simulink model "gm_soc_dvbs2_fpga"  (R2025b)
settings: Solver=VariableStepAuto  StartTime=0.0  StopTime=10.0  RelTol=1e-3
InitFcn:
  | soc_dvbs2_init;
undefined symbols (not defined in the file or in its folder): Add, coefficientsLog, coefficientsSqrt1, coefficientsSqrt2, dataBits, Deinterleaver, designMultirateFIR, noisePow, Shift, Short, soc_dvbs2_designFIRFilter, soc_dvbs2_txPacketBits, syncWord, txDataOut, txFiltCoeff, XData
libraries: simulink x304, hdlsllib x265, dspsigops x15, dsphdlfiltering2 x8, hdlmdlgenlib x6, dsphdlsigops2 x5, commseqgen3 x5, dsphdlmathfun2 x3, hwlogicconnlib x2, whdledac x2, commhdlcrc x2, whdlutilities x1
(part 32 of 36)

== system gm_soc_dvbs2_fpga/DVBS2/DVBS2 TxRx/DVB-S2 HDL Receiver/Synchronizer and PL Header Decoder/PL Header Recovery/PL Header Decoder/ML Decoder/Get Min Index/For Each Subsystem_instance29 ==
  note: For Each
  valueIn : Inport  OutDataTypeStr=fixdt(1, 25, 15)  PortDimensions=[2]  SampleTime=2.5e-07
  idxIn : Inport  Port=2  OutDataTypeStr=fixdt(0, 6, 0)  PortDimensions=[2]  SampleTime=2.5e-07
  Delay{1..9} (9 alike) : Delay  DelayLength=double(1)  InitialCondition=0  SampleTime=2.5e-07
  Relational Operator : RelationalOperator  Operator=<  OutDataTypeStr=boolean  SampleTime=2.5e-07  InputSameDT=off
  Switch : Switch  Criteria=u2 ~= 0  Threshold="fi(0,0,1,0,\"hex\",\"0\")"  OutDataTypeStr=fixdt(1, 25, 15)  SampleTime=2.5e-07  SaturateOnIntegerOverflow=off  InputSameDT=off
  Switch1 : Switch  Criteria=u2 ~= 0  Threshold="fi(0,0,1,0,\"hex\",\"0\")"  OutDataTypeStr=fixdt(0, 6, 0)  SampleTime=2.5e-07  SaturateOnIntegerOverflow=off  InputSameDT=off
  t : Demux  Outputs=2
  t1 : Demux  Outputs=2
  ValueOut : Outport  SampleTime=2.5e-07
  idxOut : Outport  Port=2  SampleTime=2.5e-07
  wires:
  Delay8/1 -> ValueOut/1
  valueIn/1 -> Delay3/1
  idxIn/1 -> Delay1/1
  t/1 -> Delay6/1
  Switch1/1 -> Delay9/1
  t1/1 -> Relational Operator/1, Delay4/1
  Delay1/1 -> t/1
  Delay3/1 -> t1/1
  t/2 -> Delay7/1
  Delay4/1 -> Switch/1
  t1/2 -> Relational Operator/2, Delay5/1
  Relational Operator/1 -> Delay2/1
  Delay5/1 -> Switch/3
  Delay6/1 -> Switch1/1
  Delay7/1 -> Switch1/3
  Delay2/1 -> Switch/2, Switch1/2
  Switch/1 -> Delay8/1
  Delay9/1 -> idxOut/1

== system gm_soc_dvbs2_fpga/DVBS2/DVBS2 TxRx/DVB-S2 HDL Receiver/Synchronizer and PL Header Decoder/PL Header Recovery/PL Header Decoder/ML Decoder/Get Min Index/For Each Subsystem_instance3 ==
  note: For Each
  valueIn : Inport  OutDataTypeStr=fixdt(1, 25, 15)  PortDimensions=[2]  SampleTime=2.5e-07
  idxIn : Inport  Port=2  OutDataTypeStr=fixdt(0, 6, 0)  PortDimensions=[2]  SampleTime=2.5e-07
  Delay{1..9} (9 alike) : Delay  DelayLength=double(1)  InitialCondition=0  SampleTime=2.5e-07
  Relational Operator : RelationalOperator  Operator=<  OutDataTypeStr=boolean  SampleTime=2.5e-07  InputSameDT=off
  Switch : Switch  Criteria=u2 ~= 0  Threshold="fi(0,0,1,0,\"hex\",\"0\")"  OutDataTypeStr=fixdt(1, 25, 15)  SampleTime=2.5e-07  SaturateOnIntegerOverflow=off  InputSameDT=off
  Switch1 : Switch  Criteria=u2 ~= 0  Threshold="fi(0,0,1,0,\"hex\",\"0\")"  OutDataTypeStr=fixdt(0, 6, 0)  SampleTime=2.5e-07  SaturateOnIntegerOverflow=off  InputSameDT=off
  t : Demux  Outputs=2
  t1 : Demux  Outputs=2
  ValueOut : Outport  SampleTime=2.5e-07
  idxOut : Outport  Port=2  SampleTime=2.5e-07
  wires:
  Delay8/1 -> ValueOut/1
  valueIn/1 -> Delay3/1
  idxIn/1 -> Delay1/1
  t/1 -> Delay6/1
  Switch1/1 -> Delay9/1
  t1/1 -> Delay4/1, Relational Operator/1
  Delay1/1 -> t/1
  Delay3/1 -> t1/1
  t/2 -> Delay7/1
  t1/2 -> Relational Operator/2, Delay5/1
  Relational Operator/1 -> Delay2/1
  Delay5/1 -> Switch/3
  Delay6/1 -> Switch1/1
  Delay7/1 -> Switch1/3
  Delay2/1 -> Switch/2, Switch1/2
  Delay4/1 -> Switch/1
  Switch/1 -> Delay8/1
  Delay9/1 -> idxOut/1

== system gm_soc_dvbs2_fpga/DVBS2/DVBS2 TxRx/DVB-S2 HDL Receiver/Synchronizer and PL Header Decoder/PL Header Recovery/PL Header Decoder/ML Decoder/Get Min Index/For Each Subsystem_instance30 ==
  note: For Each
  valueIn : Inport  OutDataTypeStr=fixdt(1, 25, 15)  PortDimensions=[2]  SampleTime=2.5e-07
  idxIn : Inport  Port=2  OutDataTypeStr=fixdt(0, 6, 0)  PortDimensions=[2]  SampleTime=2.5e-07
  Delay{1..9} (9 alike) : Delay  DelayLength=double(1)  InitialCondition=0  SampleTime=2.5e-07
  Relational Operator : RelationalOperator  Operator=<  OutDataTypeStr=boolean  SampleTime=2.5e-07  InputSameDT=off
  Switch : Switch  Criteria=u2 ~= 0  Threshold="fi(0,0,1,0,\"hex\",\"0\")"  OutDataTypeStr=fixdt(1, 25, 15)  SampleTime=2.5e-07  SaturateOnIntegerOverflow=off  InputSameDT=off
  Switch1 : Switch  Criteria=u2 ~= 0  Threshold="fi(0,0,1,0,\"hex\",\"0\")"  OutDataTypeStr=fixdt(0, 6, 0)  SampleTime=2.5e-07  SaturateOnIntegerOverflow=off  InputSameDT=off
  t : Demux  Outputs=2
  t1 : Demux  Outputs=2
  ValueOut : Outport  SampleTime=2.5e-07
  idxOut : Outport  Port=2  SampleTime=2.5e-07
  wires:
  valueIn/1 -> Delay3/1
  idxIn/1 -> Delay1/1
  Delay9/1 -> idxOut/1
  Delay1/1 -> t/1
  Delay3/1 -> t1/1
  t/1 -> Delay6/1
  t1/1 -> Relational Operator/1, Delay4/1
  t/2 -> Delay7/1
  t1/2 -> Relational Operator/2, Delay5/1
  Relational Operator/1 -> Delay2/1
  Delay5/1 -> Switch/3
  Delay6/1 -> Switch1/1
  Switch1/1 -> Delay9/1
  Delay7/1 -> Switch1/3
  Delay2/1 -> Switch1/2, Switch/2
  Delay4/1 -> Switch/1
  Delay8/1 -> ValueOut/1
  Switch/1 -> Delay8/1

== system gm_soc_dvbs2_fpga/DVBS2/DVBS2 TxRx/DVB-S2 HDL Receiver/Synchronizer and PL Header Decoder/PL Header Recovery/PL Header Decoder/ML Decoder/Get Min Index/For Each Subsystem_instance31 ==
  note: For Each
  valueIn : Inport  OutDataTypeStr=fixdt(1, 25, 15)  PortDimensions=[2]  SampleTime=2.5e-07
  idxIn : Inport  Port=2  OutDataTypeStr=fixdt(0, 6, 0)  PortDimensions=[2]  SampleTime=2.5e-07
  Delay{1..9} (9 alike) : Delay  DelayLength=double(1)  InitialCondition=0  SampleTime=2.5e-07
  Relational Operator : RelationalOperator  Operator=<  OutDataTypeStr=boolean  SampleTime=2.5e-07  InputSameDT=off
  Switch : Switch  Criteria=u2 ~= 0  Threshold="fi(0,0,1,0,\"hex\",\"0\")"  OutDataTypeStr=fixdt(1, 25, 15)  SampleTime=2.5e-07  SaturateOnIntegerOverflow=off  InputSameDT=off
  Switch1 : Switch  Criteria=u2 ~= 0  Threshold="fi(0,0,1,0,\"hex\",\"0\")"  OutDataTypeStr=fixdt(0, 6, 0)  SampleTime=2.5e-07  SaturateOnIntegerOverflow=off  InputSameDT=off
  t : Demux  Outputs=2
  t1 : Demux  Outputs=2
  ValueOut : Outport  SampleTime=2.5e-07
  idxOut : Outport  Port=2  SampleTime=2.5e-07
  wires:
  Delay8/1 -> ValueOut/1
  valueIn/1 -> Delay3/1
  Delay1/1 -> t/1
  Switch1/1 -> Delay9/1
  t1/1 -> Relational Operator/1, Delay4/1
  Delay3/1 -> t1/1
  idxIn/1 -> Delay1/1
  Relational Operator/1 -> Delay2/1
  t1/2 -> Delay5/1, Relational Operator/2
  Delay4/1 -> Switch/1
  t/1 -> Delay6/1
  t/2 -> Delay7/1
  Delay5/1 -> Switch/3
  Delay2/1 -> Switch/2, Switch1/2
  Delay6/1 -> Switch1/1
  Delay7/1 -> Switch1/3
  Switch/1 -> Delay8/1
  Delay9/1 -> idxOut/1

== system gm_soc_dvbs2_fpga/DVBS2/DVBS2 TxRx/DVB-S2 HDL Receiver/Synchronizer and PL Header Decoder/PL Header Recovery/PL Header Decoder/ML Decoder/Get Min Index/For Each Subsystem_instance32 ==
  note: For Each
  valueIn : Inport  OutDataTypeStr=fixdt(1, 25, 15)  PortDimensions=[2]  SampleTime=2.5e-07
  idxIn : Inport  Port=2  OutDataTypeStr=fixdt(0, 6, 0)  PortDimensions=[2]  SampleTime=2.5e-07
  Delay{1..9} (9 alike) : Delay  DelayLength=double(1)  InitialCondition=0  SampleTime=2.5e-07
  Relational Operator : RelationalOperator  Operator=<  OutDataTypeStr=boolean  SampleTime=2.5e-07  InputSameDT=off
  Switch : Switch  Criteria=u2 ~= 0  Threshold="fi(0,0,1,0,\"hex\",\"0\")"  OutDataTypeStr=fixdt(1, 25, 15)  SampleTime=2.5e-07  SaturateOnIntegerOverflow=off  InputSameDT=off
  Switch1 : Switch  Criteria=u2 ~= 0  Threshold="fi(0,0,1,0,\"hex\",\"0\")"  OutDataTypeStr=fixdt(0, 6, 0)  SampleTime=2.5e-07  SaturateOnIntegerOverflow=off  InputSameDT=off
  t : Demux  Outputs=2
  t1 : Demux  Outputs=2
  ValueOut : Outport  SampleTime=2.5e-07
  idxOut : Outport  Port=2  SampleTime=2.5e-07
  wires:
  Delay8/1 -> ValueOut/1
  valueIn/1 -> Delay3/1
  Delay1/1 -> t/1
  Switch1/1 -> Delay9/1
  t1/1 -> Relational Operator/1, Delay4/1
  Delay3/1 -> t1/1
  idxIn/1 -> Delay1/1
  Relational Operator/1 -> Delay2/1
  t1/2 -> Delay5/1, Relational Operator/2
  Delay4/1 -> Switch/1
  t/1 -> Delay6/1
  t/2 -> Delay7/1
  Delay5/1 -> Switch/3
  Delay2/1 -> Switch/2, Switch1/2
  Delay6/1 -> Switch1/1
  Delay7/1 -> Switch1/3
  Switch/1 -> Delay8/1
  Delay9/1 -> idxOut/1

== system gm_soc_dvbs2_fpga/DVBS2/DVBS2 TxRx/DVB-S2 HDL Receiver/Synchronizer and PL Header Decoder/PL Header Recovery/PL Header Decoder/ML Decoder/Get Min Index/For Each Subsystem_instance4 ==
  note: For Each
  valueIn : Inport  OutDataTypeStr=fixdt(1, 25, 15)  PortDimensions=[2]  SampleTime=2.5e-07
  idxIn : Inport  Port=2  OutDataTypeStr=fixdt(0, 6, 0)  PortDimensions=[2]  SampleTime=2.5e-07
  Delay{1..9} (9 alike) : Delay  DelayLength=double(1)  InitialCondition=0  SampleTime=2.5e-07
  Relational Operator : RelationalOperator  Operator=<  OutDataTypeStr=boolean  SampleTime=2.5e-07  InputSameDT=off
  Switch : Switch  Criteria=u2 ~= 0  Threshold="fi(0,0,1,0,\"hex\",\"0\")"  OutDataTypeStr=fixdt(1, 25, 15)  SampleTime=2.5e-07  SaturateOnIntegerOverflow=off  InputSameDT=off
  Switch1 : Switch  Criteria=u2 ~= 0  Threshold="fi(0,0,1,0,\"hex\",\"0\")"  OutDataTypeStr=fixdt(0, 6, 0)  SampleTime=2.5e-07  SaturateOnIntegerOverflow=off  InputSameDT=off
  t : Demux  Outputs=2
  t1 : Demux  Outputs=2
  ValueOut : Outport  SampleTime=2.5e-07
  idxOut : Outport  Port=2  SampleTime=2.5e-07
  wires:
  Delay8/1 -> ValueOut/1
  valueIn/1 -> Delay3/1
  idxIn/1 -> Delay1/1
  t/1 -> Delay6/1
  Switch1/1 -> Delay9/1
  t1/1 -> Delay4/1, Relational Operator/1
  Delay1/1 -> t/1
  Delay3/1 -> t1/1
  t/2 -> Delay7/1
  Delay4/1 -> Switch/1
  t1/2 -> Relational Operator/2, Delay5/1
  Relational Operator/1 -> Delay2/1
  Delay5/1 -> Switch/3
  Delay6/1 -> Switch1/1
  Delay7/1 -> Switch1/3
  Delay2/1 -> Switch/2, Switch1/2
  Switch/1 -> Delay8/1
  Delay9/1 -> idxOut/1

== system gm_soc_dvbs2_fpga/DVBS2/DVBS2 TxRx/DVB-S2 HDL Receiver/Synchronizer and PL Header Decoder/PL Header Recovery/PL Header Decoder/ML Decoder/Get Min Index/For Each Subsystem_instance5 ==
  note: For Each
  valueIn : Inport  OutDataTypeStr=fixdt(1, 25, 15)  PortDimensions=[2]  SampleTime=2.5e-07
  idxIn : Inport  Port=2  OutDataTypeStr=fixdt(0, 6, 0)  PortDimensions=[2]  SampleTime=2.5e-07
  Delay{1..9} (9 alike) : Delay  DelayLength=double(1)  InitialCondition=0  SampleTime=2.5e-07
  Relational Operator : RelationalOperator  Operator=<  OutDataTypeStr=boolean  SampleTime=2.5e-07  InputSameDT=off
  Switch : Switch  Criteria=u2 ~= 0  Threshold="fi(0,0,1,0,\"hex\",\"0\")"  OutDataTypeStr=fixdt(1, 25, 15)  SampleTime=2.5e-07  SaturateOnIntegerOverflow=off  InputSameDT=off
  Switch1 : Switch  Criteria=u2 ~= 0  Threshold="fi(0,0,1,0,\"hex\",\"0\")"  OutDataTypeStr=fixdt(0, 6, 0)  SampleTime=2.5e-07  SaturateOnIntegerOverflow=off  InputSameDT=off
  t : Demux  Outputs=2
  t1 : Demux  Outputs=2
  ValueOut : Outport  SampleTime=2.5e-07
  idxOut : Outport  Port=2  SampleTime=2.5e-07
  wires:
  valueIn/1 -> Delay3/1
  idxIn/1 -> Delay1/1
  Delay9/1 -> idxOut/1
  Delay1/1 -> t/1
  Delay3/1 -> t1/1
  t/1 -> Delay6/1
  t1/1 -> Delay4/1, Relational Operator/1
  t/2 -> Delay7/1
  t1/2 -> Relational Operator/2, Delay5/1
  Relational Operator/1 -> Delay2/1
  Delay5/1 -> Switch/3
  Delay6/1 -> Switch1/1
  Switch1/1 -> Delay9/1
  Delay7/1 -> Switch1/3
  Delay2/1 -> Switch/2, Switch1/2
  Delay4/1 -> Switch/1
  Switch/1 -> Delay8/1
  Delay8/1 -> ValueOut/1

== system gm_soc_dvbs2_fpga/DVBS2/DVBS2 TxRx/DVB-S2 HDL Receiver/Synchronizer and PL Header Decoder/PL Header Recovery/PL Header Decoder/ML Decoder/Get Min Index/For Each Subsystem_instance6 ==
  note: For Each
  valueIn : Inport  OutDataTypeStr=fixdt(1, 25, 15)  PortDimensions=[2]  SampleTime=2.5e-07
  idxIn : Inport  Port=2  OutDataTypeStr=fixdt(0, 6, 0)  PortDimensions=[2]  SampleTime=2.5e-07
  Delay{1..9} (9 alike) : Delay  DelayLength=double(1)  InitialCondition=0  SampleTime=2.5e-07
  Relational Operator : RelationalOperator  Operator=<  OutDataTypeStr=boolean  SampleTime=2.5e-07  InputSameDT=off
  Switch : Switch  Criteria=u2 ~= 0  Threshold="fi(0,0,1,0,\"hex\",\"0\")"  OutDataTypeStr=fixdt(1, 25, 15)  SampleTime=2.5e-07  SaturateOnIntegerOverflow=off  InputSameDT=off
  Switch1 : Switch  Criteria=u2 ~= 0  Threshold="fi(0,0,1,0,\"hex\",\"0\")"  OutDataTypeStr=fixdt(0, 6, 0)  SampleTime=2.5e-07  SaturateOnIntegerOverflow=off  InputSameDT=off
  t : Demux  Outputs=2
  t1 : Demux  Outputs=2
  ValueOut : Outport  SampleTime=2.5e-07
  idxOut : Outport  Port=2  SampleTime=2.5e-07
  wires:
  Delay8/1 -> ValueOut/1
  valueIn/1 -> Delay3/1
  idxIn/1 -> Delay1/1
  t/1 -> Delay6/1
  Switch1/1 -> Delay9/1
  t1/1 -> Delay4/1, Relational Operator/1
  Delay1/1 -> t/1
  Delay3/1 -> t1/1
  t/2 -> Delay7/1
  Delay4/1 -> Switch/1
  t1/2 -> Delay5/1, Relational Operator/2
  Relational Operator/1 -> Delay2/1
  Delay5/1 -> Switch/3
  Delay6/1 -> Switch1/1
  Delay7/1 -> Switch1/3
  Delay2/1 -> Switch/2, Switch1/2
  Switch/1 -> Delay8/1
  Delay9/1 -> idxOut/1

== system gm_soc_dvbs2_fpga/DVBS2/DVBS2 TxRx/DVB-S2 HDL Receiver/Synchronizer and PL Header Decoder/PL Header Recovery/PL Header Decoder/ML Decoder/Get Min Index/For Each Subsystem_instance7 ==
  note: For Each
  valueIn : Inport  OutDataTypeStr=fixdt(1, 25, 15)  PortDimensions=[2]  SampleTime=2.5e-07
  idxIn : Inport  Port=2  OutDataTypeStr=fixdt(0, 6, 0)  PortDimensions=[2]  SampleTime=2.5e-07
  Delay{1..9} (9 alike) : Delay  DelayLength=double(1)  InitialCondition=0  SampleTime=2.5e-07
  Relational Operator : RelationalOperator  Operator=<  OutDataTypeStr=boolean  SampleTime=2.5e-07  InputSameDT=off
  Switch : Switch  Criteria=u2 ~= 0  Threshold="fi(0,0,1,0,\"hex\",\"0\")"  OutDataTypeStr=fixdt(1, 25, 15)  SampleTime=2.5e-07  SaturateOnIntegerOverflow=off  InputSameDT=off
  Switch1 : Switch  Criteria=u2 ~= 0  Threshold="fi(0,0,1,0,\"hex\",\"0\")"  OutDataTypeStr=fixdt(0, 6, 0)  SampleTime=2.5e-07  SaturateOnIntegerOverflow=off  InputSameDT=off
  t : Demux  Outputs=2
  t1 : Demux  Outputs=2
  ValueOut : Outport  SampleTime=2.5e-07
  idxOut : Outport  Port=2  SampleTime=2.5e-07
  wires:
  Delay8/1 -> ValueOut/1
  valueIn/1 -> Delay3/1
  Delay1/1 -> t/1
  Switch1/1 -> Delay9/1
  t1/1 -> Relational Operator/1, Delay4/1
  Delay3/1 -> t1/1
  idxIn/1 -> Delay1/1
  Relational Operator/1 -> Delay2/1
  t1/2 -> Delay5/1, Relational Operator/2
  Delay4/1 -> Switch/1
  t/1 -> Delay6/1
  t/2 -> Delay7/1
  Delay5/1 -> Switch/3
  Delay2/1 -> Switch/2, Switch1/2
  Delay6/1 -> Switch1/1
  Delay7/1 -> Switch1/3
  Switch/1 -> Delay8/1
  Delay9/1 -> idxOut/1

== system gm_soc_dvbs2_fpga/DVBS2/DVBS2 TxRx/DVB-S2 HDL Receiver/Synchronizer and PL Header Decoder/PL Header Recovery/PL Header Decoder/ML Decoder/Get Min Index/For Each Subsystem_instance8 ==
  note: For Each
  valueIn : Inport  OutDataTypeStr=fixdt(1, 25, 15)  PortDimensions=[2]  SampleTime=2.5e-07
  idxIn : Inport  Port=2  OutDataTypeStr=fixdt(0, 6, 0)  PortDimensions=[2]  SampleTime=2.5e-07
  Delay{1..9} (9 alike) : Delay  DelayLength=double(1)  InitialCondition=0  SampleTime=2.5e-07
  Relational Operator : RelationalOperator  Operator=<  OutDataTypeStr=boolean  SampleTime=2.5e-07  InputSameDT=off
  Switch : Switch  Criteria=u2 ~= 0  Threshold="fi(0,0,1,0,\"hex\",\"0\")"  OutDataTypeStr=fixdt(1, 25, 15)  SampleTime=2.5e-07  SaturateOnIntegerOverflow=off  InputSameDT=off
  Switch1 : Switch  Criteria=u2 ~= 0  Threshold="fi(0,0,1,0,\"hex\",\"0\")"  OutDataTypeStr=fixdt(0, 6, 0)  SampleTime=2.5e-07  SaturateOnIntegerOverflow=off  InputSameDT=off
  t : Demux  Outputs=2
  t1 : Demux  Outputs=2
  ValueOut : Outport  SampleTime=2.5e-07
  idxOut : Outport  Port=2  SampleTime=2.5e-07
  wires:
  valueIn/1 -> Delay3/1
  Delay9/1 -> idxOut/1
  Delay1/1 -> t/1
  idxIn/1 -> Delay1/1
  Delay3/1 -> t1/1
  Switch1/1 -> Delay9/1
  t1/1 -> Relational Operator/1, Delay4/1
  Relational Operator/1 -> Delay2/1
  t1/2 -> Delay5/1, Relational Operator/2
  Delay4/1 -> Switch/1
  t/1 -> Delay6/1
  t/2 -> Delay7/1
  Delay5/1 -> Switch/3
  Delay2/1 -> Switch/2, Switch1/2
  Delay6/1 -> Switch1/1
  Delay7/1 -> Switch1/3
  Switch/1 -> Delay8/1
  Delay8/1 -> ValueOut/1

== system gm_soc_dvbs2_fpga/DVBS2/DVBS2 TxRx/DVB-S2 HDL Receiver/Synchronizer and PL Header Decoder/PL Header Recovery/PL Header Decoder/ML Decoder/Get Min Index/For Each Subsystem_instance9 ==
  note: For Each
  valueIn : Inport  OutDataTypeStr=fixdt(1, 25, 15)  PortDimensions=[2]  SampleTime=2.5e-07
  idxIn : Inport  Port=2  OutDataTypeStr=fixdt(0, 6, 0)  PortDimensions=[2]  SampleTime=2.5e-07
  Delay{1..9} (9 alike) : Delay  DelayLength=double(1)  InitialCondition=0  SampleTime=2.5e-07
  Relational Operator : RelationalOperator  Operator=<  OutDataTypeStr=boolean  SampleTime=2.5e-07  InputSameDT=off
  Switch : Switch  Criteria=u2 ~= 0  Threshold="fi(0,0,1,0,\"hex\",\"0\")"  OutDataTypeStr=fixdt(1, 25, 15)  SampleTime=2.5e-07  SaturateOnIntegerOverflow=off  InputSameDT=off
  Switch1 : Switch  Criteria=u2 ~= 0  Threshold="fi(0,0,1,0,\"hex\",\"0\")"  OutDataTypeStr=fixdt(0, 6, 0)  SampleTime=2.5e-07  SaturateOnIntegerOverflow=off  InputSameDT=off
  t : Demux  Outputs=2
  t1 : Demux  Outputs=2
  ValueOut : Outport  SampleTime=2.5e-07
  idxOut : Outport  Port=2  SampleTime=2.5e-07
  wires:
  Delay8/1 -> ValueOut/1
  valueIn/1 -> Delay3/1
  Delay1/1 -> t/1
  Switch1/1 -> Delay9/1
  t1/1 -> Relational Operator/1, Delay4/1
  Delay3/1 -> t1/1
  idxIn/1 -> Delay1/1
  Relational Operator/1 -> Delay2/1
  t1/2 -> Delay5/1, Relational Operator/2
  Delay4/1 -> Switch/1
  t/1 -> Delay6/1
  t/2 -> Delay7/1
  Delay5/1 -> Switch/3
  Delay2/1 -> Switch/2, Switch1/2
  Delay6/1 -> Switch1/1
  Delay7/1 -> Switch1/3
  Switch/1 -> Delay8/1
  Delay9/1 -> idxOut/1

== system gm_soc_dvbs2_fpga/DVBS2/DVBS2 TxRx/DVB-S2 HDL Receiver/Synchronizer and PL Header Decoder/PL Header Recovery/PL Header Decoder/ML Decoder/Integer to Bit Convertor/For Each Subsystem1_instance1 ==
  note: For Each
  In1 : Inport  OutDataTypeStr=uint8  PortDimensions=1  SampleTime=2.5e-07
  Extract Bits2 : simulink/Logic and Bit Operations/Extract Bits  bitsToExtract=Upper half  numBits=8  bitIdxRange=[32 63]  outScalingMode=Treat bit field as an integer
  Extract Bits3 : simulink/Logic and Bit Operations/Extract Bits  bitsToExtract=Lower half  numBits=8  bitIdxRange=[32 63]  outScalingMode=Treat bit field as an integer
  Mux1 : Mux  Inputs=2
  Out1 : Outport  SampleTime=2.5e-07
  wires:
  In1/1 -> Extract Bits2/1, Extract Bits3/1
  Extract Bits3/1 -> Mux1/2
  Extract Bits2/1 -> Mux1/1
  Mux1/1 -> Out1/1

== system gm_soc_dvbs2_fpga/DVBS2/DVBS2 TxRx/DVB-S2 HDL Receiver/Synchronizer and PL Header Decoder/PL Header Recovery/PL Header Decoder/ML Decoder/Integer to Bit Convertor/For Each Subsystem1_instance2 ==
  note: For Each
  In1 : Inport  OutDataTypeStr=uint8  PortDimensions=1  SampleTime=2.5e-07
  Extract Bits2 : simulink/Logic and Bit Operations/Extract Bits  bitsToExtract=Upper half  numBits=8  bitIdxRange=[32 63]  outScalingMode=Treat bit field as an integer
  Extract Bits3 : simulink/Logic and Bit Operations/Extract Bits  bitsToExtract=Lower half  numBits=8  bitIdxRange=[32 63]  outScalingMode=Treat bit field as an integer
  Mux1 : Mux  Inputs=2
  Out1 : Outport  SampleTime=2.5e-07
  wires:
  Extract Bits3/1 -> Mux1/2
  In1/1 -> Extract Bits2/1, Extract Bits3/1
  Extract Bits2/1 -> Mux1/1
  Mux1/1 -> Out1/1

== system gm_soc_dvbs2_fpga/DVBS2/DVBS2 TxRx/DVB-S2 HDL Receiver/Synchronizer and PL Header Decoder/PL Header Recovery/PL Header Decoder/ML Decoder/Integer to Bit Convertor/For Each Subsystem1_instance3 ==
  note: For Each
  In1 : Inport  OutDataTypeStr=uint8  PortDimensions=1  SampleTime=2.5e-07
  Extract Bits2 : simulink/Logic and Bit Operations/Extract Bits  bitsToExtract=Upper half  numBits=8  bitIdxRange=[32 63]  outScalingMode=Treat bit field as an integer
  Extract Bits3 : simulink/Logic and Bit Operations/Extract Bits  bitsToExtract=Lower half  numBits=8  bitIdxRange=[32 63]  outScalingMode=Treat bit field as an integer
  Mux1 : Mux  Inputs=2
  Out1 : Outport  SampleTime=2.5e-07
  wires:
  In1/1 -> Extract Bits2/1, Extract Bits3/1
  Extract Bits3/1 -> Mux1/2
  Extract Bits2/1 -> Mux1/1
  Mux1/1 -> Out1/1

== system gm_soc_dvbs2_fpga/DVBS2/DVBS2 TxRx/DVB-S2 HDL Receiver/Synchronizer and PL Header Decoder/PL Header Recovery/PL Header Decoder/ML Decoder/Integer to Bit Convertor/For Each Subsystem1_instance4 ==
  note: For Each
  In1 : Inport  OutDataTypeStr=uint8  PortDimensions=1  SampleTime=2.5e-07
  Extract Bits2 : simulink/Logic and Bit Operations/Extract Bits  bitsToExtract=Upper half  numBits=8  bitIdxRange=[32 63]  outScalingMode=Treat bit field as an integer
  Extract Bits3 : simulink/Logic and Bit Operations/Extract Bits  bitsToExtract=Lower half  numBits=8  bitIdxRange=[32 63]  outScalingMode=Treat bit field as an integer
  Mux1 : Mux  Inputs=2
  Out1 : Outport  SampleTime=2.5e-07
  wires:
  In1/1 -> Extract Bits2/1, Extract Bits3/1
  Extract Bits2/1 -> Mux1/1
  Extract Bits3/1 -> Mux1/2
  Mux1/1 -> Out1/1

== system gm_soc_dvbs2_fpga/DVBS2/DVBS2 TxRx/DVB-S2 HDL Receiver/Synchronizer and PL Header Decoder/PL Header Recovery/PL Header Decoder/ML Decoder/Integer to Bit Convertor/For Each Subsystem2_instance1 ==
  note: For Each
  In1 : Inport  OutDataTypeStr=fixdt(0, 4, 0)  PortDimensions=1  SampleTime=2.5e-07
  Extract Bits2 : simulink/Logic and Bit Operations/Extract Bits  bitsToExtract=Upper half  numBits=8  bitIdxRange=[32 63]  outScalingMode=Treat bit field as an integer
  Extract Bits3 : simulink/Logic and Bit Operations/Extract Bits  bitsToExtract=Lower half  numBits=8  bitIdxRange=[32 63]  outScalingMode=Treat bit field as an integer
  Mux1 : Mux  Inputs=2
  Out1 : Outport  SampleTime=2.5e-07
  wires:
  In1/1 -> Extract Bits2/1, Extract Bits3/1
  Extract Bits3/1 -> Mux1/2
  Extract Bits2/1 -> Mux1/1
  Mux1/1 -> Out1/1

== system gm_soc_dvbs2_fpga/DVBS2/DVBS2 TxRx/DVB-S2 HDL Receiver/Synchronizer and PL Header Decoder/PL Header Recovery/PL Header Decoder/ML Decoder/Integer to Bit Convertor/For Each Subsystem2_instance2 ==
  note: For Each
  In1 : Inport  OutDataTypeStr=fixdt(0, 4, 0)  PortDimensions=1  SampleTime=2.5e-07
  Extract Bits2 : simulink/Logic and Bit Operations/Extract Bits  bitsToExtract=Upper half  numBits=8  bitIdxRange=[32 63]  outScalingMode=Treat bit field as an integer
  Extract Bits3 : simulink/Logic and Bit Operations/Extract Bits  bitsToExtract=Lower half  numBits=8  bitIdxRange=[32 63]  outScalingMode=Treat bit field as an integer
  Mux1 : Mux  Inputs=2
  Out1 : Outport  SampleTime=2.5e-07
  wires:
  Extract Bits3/1 -> Mux1/2
  In1/1 -> Extract Bits2/1, Extract Bits3/1
  Extract Bits2/1 -> Mux1/1
  Mux1/1 -> Out1/1

== system gm_soc_dvbs2_fpga/DVBS2/DVBS2 TxRx/DVB-S2 HDL Receiver/Synchronizer and PL Header Decoder/PL Header Recovery/PL Header Decoder/ML Decoder/Integer to Bit Convertor/For Each Subsystem2_instance3 ==
  note: For Each
  In1 : Inport  OutDataTypeStr=fixdt(0, 4, 0)  PortDimensions=1  SampleTime=2.5e-07
  Extract Bits2 : simulink/Logic and Bit Operations/Extract Bits  bitsToExtract=Upper half  numBits=8  bitIdxRange=[32 63]  outScalingMode=Treat bit field as an integer
  Extract Bits3 : simulink/Logic and Bit Operations/Extract Bits  bitsToExtract=Lower half  numBits=8  bitIdxRange=[32 63]  outScalingMode=Treat bit field as an integer
  Mux1 : Mux  Inputs=2
  Out1 : Outport  SampleTime=2.5e-07
  wires:
  In1/1 -> Extract Bits2/1, Extract Bits3/1
  Extract Bits3/1 -> Mux1/2
  Extract Bits2/1 -> Mux1/1
  Mux1/1 -> Out1/1

== system gm_soc_dvbs2_fpga/DVBS2/DVBS2 TxRx/DVB-S2 HDL Receiver/Synchronizer and PL Header Decoder/PL Header Recovery/PL Header Decoder/ML Decoder/Integer to Bit Convertor/For Each Subsystem2_instance4 ==
  note: For Each
  In1 : Inport  OutDataTypeStr=fixdt(0, 4, 0)  PortDimensions=1  SampleTime=2.5e-07
  Extract Bits2 : simulink/Logic and Bit Operations/Extract Bits  bitsToExtract=Upper half  numBits=8  bitIdxRange=[32 63]  outScalingMode=Treat bit field as an integer
  Extract Bits3 : simulink/Logic and Bit Operations/Extract Bits  bitsToExtract=Lower half  numBits=8  bitIdxRange=[32 63]  outScalingMode=Treat bit field as an integer
  Mux1 : Mux  Inputs=2
  Out1 : Outport  SampleTime=2.5e-07
  wires:
  In1/1 -> Extract Bits2/1, Extract Bits3/1
  Extract Bits2/1 -> Mux1/1
  Extract Bits3/1 -> Mux1/2
  Mux1/1 -> Out1/1

== system gm_soc_dvbs2_fpga/DVBS2/DVBS2 TxRx/DVB-S2 HDL Receiver/Synchronizer and PL Header Decoder/PL Header Recovery/PL Header Decoder/ML Decoder/Integer to Bit Convertor/For Each Subsystem2_instance5 ==
  note: For Each
  In1 : Inport  OutDataTypeStr=fixdt(0, 4, 0)  PortDimensions=1  SampleTime=2.5e-07
  Extract Bits2 : simulink/Logic and Bit Operations/Extract Bits  bitsToExtract=Upper half  numBits=8  bitIdxRange=[32 63]  outScalingMode=Treat bit field as an integer
  Extract Bits3 : simulink/Logic and Bit Operations/Extract Bits  bitsToExtract=Lower half  numBits=8  bitIdxRange=[32 63]  outScalingMode=Treat bit field as an integer
  Mux1 : Mux  Inputs=2
  Out1 : Outport  SampleTime=2.5e-07
  wires:
  Extract Bits3/1 -> Mux1/2
  In1/1 -> Extract Bits2/1, Extract Bits3/1
  Extract Bits2/1 -> Mux1/1
  Mux1/1 -> Out1/1

== system gm_soc_dvbs2_fpga/DVBS2/DVBS2 TxRx/DVB-S2 HDL Receiver/Synchronizer and PL Header Decoder/PL Header Recovery/PL Header Decoder/ML Decoder/Integer to Bit Convertor/For Each Subsystem2_instance6 ==
  note: For Each
  In1 : Inport  OutDataTypeStr=fixdt(0, 4, 0)  PortDimensions=1  SampleTime=2.5e-07
  Extract Bits2 : simulink/Logic and Bit Operations/Extract Bits  bitsToExtract=Upper half  numBits=8  bitIdxRange=[32 63]  outScalingMode=Treat bit field as an integer
  Extract Bits3 : simulink/Logic and Bit Operations/Extract Bits  bitsToExtract=Lower half  numBits=8  bitIdxRange=[32 63]  outScalingMode=Treat bit field as an integer
  Mux1 : Mux  Inputs=2
  Out1 : Outport  SampleTime=2.5e-07
  wires:
  In1/1 -> Extract Bits2/1, Extract Bits3/1
  Extract Bits3/1 -> Mux1/2
  Extract Bits2/1 -> Mux1/1
  Mux1/1 -> Out1/1

== system gm_soc_dvbs2_fpga/DVBS2/DVBS2 TxRx/DVB-S2 HDL Receiver/Synchronizer and PL Header Decoder/PL Header Recovery/PL Header Decoder/ML Decoder/Integer to Bit Convertor/For Each Subsystem2_instance7 ==
  note: For Each
  In1 : Inport  OutDataTypeStr=fixdt(0, 4, 0)  PortDimensions=1  SampleTime=2.5e-07
  Extract Bits2 : simulink/Logic and Bit Operations/Extract Bits  bitsToExtract=Upper half  numBits=8  bitIdxRange=[32 63]  outScalingMode=Treat bit field as an integer
  Extract Bits3 : simulink/Logic and Bit Operations/Extract Bits  bitsToExtract=Lower half  numBits=8  bitIdxRange=[32 63]  outScalingMode=Treat bit field as an integer
  Mux1 : Mux  Inputs=2
  Out1 : Outport  SampleTime=2.5e-07
  wires:
  Extract Bits3/1 -> Mux1/2
  In1/1 -> Extract Bits2/1, Extract Bits3/1
  Extract Bits2/1 -> Mux1/1
  Mux1/1 -> Out1/1

== system gm_soc_dvbs2_fpga/DVBS2/DVBS2 TxRx/DVB-S2 HDL Receiver/Synchronizer and PL Header Decoder/PL Header Recovery/PL Header Decoder/ML Decoder/Integer to Bit Convertor/For Each Subsystem2_instance8 ==
  note: For Each
  In1 : Inport  OutDataTypeStr=fixdt(0, 4, 0)  PortDimensions=1  SampleTime=2.5e-07
  Extract Bits2 : simulink/Logic and Bit Operations/Extract Bits  bitsToExtract=Upper half  numBits=8  bitIdxRange=[32 63]  outScalingMode=Treat bit field as an integer
  Extract Bits3 : simulink/Logic and Bit Operations/Extract Bits  bitsToExtract=Lower half  numBits=8  bitIdxRange=[32 63]  outScalingMode=Treat bit field as an integer
  Mux1 : Mux  Inputs=2
  Out1 : Outport  SampleTime=2.5e-07
  wires:
  In1/1 -> Extract Bits2/1, Extract Bits3/1
  Extract Bits3/1 -> Mux1/2
  Extract Bits2/1 -> Mux1/1
  Mux1/1 -> Out1/1

== system gm_soc_dvbs2_fpga/DVBS2/DVBS2 TxRx/DVB-S2 HDL Receiver/Synchronizer and PL Header Decoder/PL Header Recovery/PL Header Decoder/ML Decoder/Integer to Bit Convertor/For Each Subsystem3_instance1 ==
  note: For Each
  In1 : Inport  OutDataTypeStr=fixdt(0, 2, 0)  PortDimensions=1  SampleTime=2.5e-07
  Extract Bits2 : simulink/Logic and Bit Operations/Extract Bits  bitsToExtract=Upper half  numBits=8  bitIdxRange=[32 63]  outScalingMode=Treat bit field as an integer
  Extract Bits3 : simulink/Logic and Bit Operations/Extract Bits  bitsToExtract=Lower half  numBits=8  bitIdxRange=[32 63]  outScalingMode=Treat bit field as an integer
  Mux1 : Mux  Inputs=2
  Out1 : Outport  SampleTime=2.5e-07
  wires:
  In1/1 -> Extract Bits2/1, Extract Bits3/1
  Extract Bits3/1 -> Mux1/2
  Extract Bits2/1 -> Mux1/1
  Mux1/1 -> Out1/1

== system gm_soc_dvbs2_fpga/DVBS2/DVBS2 TxRx/DVB-S2 HDL Receiver/Synchronizer and PL Header Decoder/PL Header Recovery/PL Header Decoder/ML Decoder/Integer to Bit Convertor/For Each Subsystem3_instance10 ==
  note: For Each
  In1 : Inport  OutDataTypeStr=fixdt(0, 2, 0)  PortDimensions=1  SampleTime=2.5e-07
  Extract Bits2 : simulink/Logic and Bit Operations/Extract Bits  bitsToExtract=Upper half  numBits=8  bitIdxRange=[32 63]  outScalingMode=Treat bit field as an integer
  Extract Bits3 : simulink/Logic and Bit Operations/Extract Bits  bitsToExtract=Lower half  numBits=8  bitIdxRange=[32 63]  outScalingMode=Treat bit field as an integer
  Mux1 : Mux  Inputs=2
  Out1 : Outport  SampleTime=2.5e-07
  wires:
  Extract Bits3/1 -> Mux1/2
  In1/1 -> Extract Bits2/1, Extract Bits3/1
  Extract Bits2/1 -> Mux1/1
  Mux1/1 -> Out1/1

== system gm_soc_dvbs2_fpga/DVBS2/DVBS2 TxRx/DVB-S2 HDL Receiver/Synchronizer and PL Header Decoder/PL Header Recovery/PL Header Decoder/ML Decoder/Integer to Bit Convertor/For Each Subsystem3_instance11 ==
  note: For Each
  In1 : Inport  OutDataTypeStr=fixdt(0, 2, 0)  PortDimensions=1  SampleTime=2.5e-07
  Extract Bits2 : simulink/Logic and Bit Operations/Extract Bits  bitsToExtract=Upper half  numBits=8  bitIdxRange=[32 63]  outScalingMode=Treat bit field as an integer
  Extract Bits3 : simulink/Logic and Bit Operations/Extract Bits  bitsToExtract=Lower half  numBits=8  bitIdxRange=[32 63]  outScalingMode=Treat bit field as an integer
  Mux1 : Mux  Inputs=2
  Out1 : Outport  SampleTime=2.5e-07
  wires:
  In1/1 -> Extract Bits2/1, Extract Bits3/1
  Extract Bits3/1 -> Mux1/2
  Extract Bits2/1 -> Mux1/1
  Mux1/1 -> Out1/1

== system gm_soc_dvbs2_fpga/DVBS2/DVBS2 TxRx/DVB-S2 HDL Receiver/Synchronizer and PL Header Decoder/PL Header Recovery/PL Header Decoder/ML Decoder/Integer to Bit Convertor/For Each Subsystem3_instance12 ==
  note: For Each
  In1 : Inport  OutDataTypeStr=fixdt(0, 2, 0)  PortDimensions=1  SampleTime=2.5e-07
  Extract Bits2 : simulink/Logic and Bit Operations/Extract Bits  bitsToExtract=Upper half  numBits=8  bitIdxRange=[32 63]  outScalingMode=Treat bit field as an integer
  Extract Bits3 : simulink/Logic and Bit Operations/Extract Bits  bitsToExtract=Lower half  numBits=8  bitIdxRange=[32 63]  outScalingMode=Treat bit field as an integer
  Mux1 : Mux  Inputs=2
  Out1 : Outport  SampleTime=2.5e-07
  wires:
  Extract Bits3/1 -> Mux1/2
  In1/1 -> Extract Bits2/1, Extract Bits3/1
  Extract Bits2/1 -> Mux1/1
  Mux1/1 -> Out1/1

== system gm_soc_dvbs2_fpga/DVBS2/DVBS2 TxRx/DVB-S2 HDL Receiver/Synchronizer and PL Header Decoder/PL Header Recovery/PL Header Decoder/ML Decoder/Integer to Bit Convertor/For Each Subsystem3_instance13 ==
  note: For Each
  In1 : Inport  OutDataTypeStr=fixdt(0, 2, 0)  PortDimensions=1  SampleTime=2.5e-07
  Extract Bits2 : simulink/Logic and Bit Operations/Extract Bits  bitsToExtract=Upper half  numBits=8  bitIdxRange=[32 63]  outScalingMode=Treat bit field as an integer
  Extract Bits3 : simulink/Logic and Bit Operations/Extract Bits  bitsToExtract=Lower half  numBits=8  bitIdxRange=[32 63]  outScalingMode=Treat bit field as an integer
  Mux1 : Mux  Inputs=2
  Out1 : Outport  SampleTime=2.5e-07
  wires:
  Extract Bits3/1 -> Mux1/2
  In1/1 -> Extract Bits2/1, Extract Bits3/1
  Extract Bits2/1 -> Mux1/1
  Mux1/1 -> Out1/1

== system gm_soc_dvbs2_fpga/DVBS2/DVBS2 TxRx/DVB-S2 HDL Receiver/Synchronizer and PL Header Decoder/PL Header Recovery/PL Header Decoder/ML Decoder/Integer to Bit Convertor/For Each Subsystem3_instance14 ==
  note: For Each
  In1 : Inport  OutDataTypeStr=fixdt(0, 2, 0)  PortDimensions=1  SampleTime=2.5e-07
  Extract Bits2 : simulink/Logic and Bit Operations/Extract Bits  bitsToExtract=Upper half  numBits=8  bitIdxRange=[32 63]  outScalingMode=Treat bit field as an integer
  Extract Bits3 : simulink/Logic and Bit Operations/Extract Bits  bitsToExtract=Lower half  numBits=8  bitIdxRange=[32 63]  outScalingMode=Treat bit field as an integer
  Mux1 : Mux  Inputs=2
  Out1 : Outport  SampleTime=2.5e-07
  wires:
  In1/1 -> Extract Bits2/1, Extract Bits3/1
  Extract Bits3/1 -> Mux1/2
  Extract Bits2/1 -> Mux1/1
  Mux1/1 -> Out1/1

== system gm_soc_dvbs2_fpga/DVBS2/DVBS2 TxRx/DVB-S2 HDL Receiver/Synchronizer and PL Header Decoder/PL Header Recovery/PL Header Decoder/ML Decoder/Integer to Bit Convertor/For Each Subsystem3_instance15 ==
  note: For Each
  In1 : Inport  OutDataTypeStr=fixdt(0, 2, 0)  PortDimensions=1  SampleTime=2.5e-07
  Extract Bits2 : simulink/Logic and Bit Operations/Extract Bits  bitsToExtract=Upper half  numBits=8  bitIdxRange=[32 63]  outScalingMode=Treat bit field as an integer
  Extract Bits3 : simulink/Logic and Bit Operations/Extract Bits  bitsToExtract=Lower half  numBits=8  bitIdxRange=[32 63]  outScalingMode=Treat bit field as an integer
  Mux1 : Mux  Inputs=2
  Out1 : Outport  SampleTime=2.5e-07
  wires:
  Extract Bits3/1 -> Mux1/2
  In1/1 -> Extract Bits2/1, Extract Bits3/1
  Extract Bits2/1 -> Mux1/1
  Mux1/1 -> Out1/1

== system gm_soc_dvbs2_fpga/DVBS2/DVBS2 TxRx/DVB-S2 HDL Receiver/Synchronizer and PL Header Decoder/PL Header Recovery/PL Header Decoder/ML Decoder/Integer to Bit Convertor/For Each Subsystem3_instance16 ==
  note: For Each
  In1 : Inport  OutDataTypeStr=fixdt(0, 2, 0)  PortDimensions=1  SampleTime=2.5e-07
  Extract Bits2 : simulink/Logic and Bit Operations/Extract Bits  bitsToExtract=Upper half  numBits=8  bitIdxRange=[32 63]  outScalingMode=Treat bit field as an integer
  Extract Bits3 : simulink/Logic and Bit Operations/Extract Bits  bitsToExtract=Lower half  numBits=8  bitIdxRange=[32 63]  outScalingMode=Treat bit field as an integer
  Mux1 : Mux  Inputs=2
  Out1 : Outport  SampleTime=2.5e-07
  wires:
  In1/1 -> Extract Bits2/1, Extract Bits3/1
  Extract Bits3/1 -> Mux1/2
  Extract Bits2/1 -> Mux1/1
  Mux1/1 -> Out1/1

== system gm_soc_dvbs2_fpga/DVBS2/DVBS2 TxRx/DVB-S2 HDL Receiver/Synchronizer and PL Header Decoder/PL Header Recovery/PL Header Decoder/ML Decoder/Integer to Bit Convertor/For Each Subsystem3_instance2 ==
  note: For Each
  In1 : Inport  OutDataTypeStr=fixdt(0, 2, 0)  PortDimensions=1  SampleTime=2.5e-07
  Extract Bits2 : simulink/Logic and Bit Operations/Extract Bits  bitsToExtract=Upper half  numBits=8  bitIdxRange=[32 63]  outScalingMode=Treat bit field as an integer
  Extract Bits3 : simulink/Logic and Bit Operations/Extract Bits  bitsToExtract=Lower half  numBits=8  bitIdxRange=[32 63]  outScalingMode=Treat bit field as an integer
  Mux1 : Mux  Inputs=2
  Out1 : Outport  SampleTime=2.5e-07
  wires:
  In1/1 -> Extract Bits2/1, Extract Bits3/1
  Extract Bits2/1 -> Mux1/1
  Extract Bits3/1 -> Mux1/2
  Mux1/1 -> Out1/1

== system gm_soc_dvbs2_fpga/DVBS2/DVBS2 TxRx/DVB-S2 HDL Receiver/Synchronizer and PL Header Decoder/PL Header Recovery/PL Header Decoder/ML Decoder/Integer to Bit Convertor/For Each Subsystem3_instance3 ==
  note: For Each
  In1 : Inport  OutDataTypeStr=fixdt(0, 2, 0)  PortDimensions=1  SampleTime=2.5e-07
  Extract Bits2 : simulink/Logic and Bit Operations/Extract Bits  bitsToExtract=Upper half  numBits=8  bitIdxRange=[32 63]  outScalingMode=Treat bit field as an integer
  Extract Bits3 : simulink/Logic and Bit Operations/Extract Bits  bitsToExtract=Lower half  numBits=8  bitIdxRange=[32 63]  outScalingMode=Treat bit field as an integer
  Mux1 : Mux  Inputs=2
  Out1 : Outport  SampleTime=2.5e-07
  wires:
  Extract Bits3/1 -> Mux1/2
  In1/1 -> Extract Bits2/1, Extract Bits3/1
  Extract Bits2/1 -> Mux1/1
  Mux1/1 -> Out1/1

== system gm_soc_dvbs2_fpga/DVBS2/DVBS2 TxRx/DVB-S2 HDL Receiver/Synchronizer and PL Header Decoder/PL Header Recovery/PL Header Decoder/ML Decoder/Integer to Bit Convertor/For Each Subsystem3_instance4 ==
  note: For Each
  In1 : Inport  OutDataTypeStr=fixdt(0, 2, 0)  PortDimensions=1  SampleTime=2.5e-07
  Extract Bits2 : simulink/Logic and Bit Operations/Extract Bits  bitsToExtract=Upper half  numBits=8  bitIdxRange=[32 63]  outScalingMode=Treat bit field as an integer
  Extract Bits3 : simulink/Logic and Bit Operations/Extract Bits  bitsToExtract=Lower half  numBits=8  bitIdxRange=[32 63]  outScalingMode=Treat bit field as an integer
  Mux1 : Mux  Inputs=2
  Out1 : Outport  SampleTime=2.5e-07
  wires:
  In1/1 -> Extract Bits2/1, Extract Bits3/1
  Mux1/1 -> Out1/1
  Extract Bits3/1 -> Mux1/2
  Extract Bits2/1 -> Mux1/1

== system gm_soc_dvbs2_fpga/DVBS2/DVBS2 TxRx/DVB-S2 HDL Receiver/Synchronizer and PL Header Decoder/PL Header Recovery/PL Header Decoder/ML Decoder/Integer to Bit Convertor/For Each Subsystem3_instance5 ==
  note: For Each
  In1 : Inport  OutDataTypeStr=fixdt(0, 2, 0)  PortDimensions=1  SampleTime=2.5e-07
  Extract Bits2 : simulink/Logic and Bit Operations/Extract Bits  bitsToExtract=Upper half  numBits=8  bitIdxRange=[32 63]  outScalingMode=Treat bit field as an integer
  Extract Bits3 : simulink/Logic and Bit Operations/Extract Bits  bitsToExtract=Lower half  numBits=8  bitIdxRange=[32 63]  outScalingMode=Treat bit field as an integer
  Mux1 : Mux  Inputs=2
  Out1 : Outport  SampleTime=2.5e-07
  wires:
  Extract Bits3/1 -> Mux1/2
  In1/1 -> Extract Bits2/1, Extract Bits3/1
  Extract Bits2/1 -> Mux1/1
  Mux1/1 -> Out1/1

== system gm_soc_dvbs2_fpga/DVBS2/DVBS2 TxRx/DVB-S2 HDL Receiver/Synchronizer and PL Header Decoder/PL Header Recovery/PL Header Decoder/ML Decoder/Integer to Bit Convertor/For Each Subsystem3_instance6 ==
  note: For Each
  In1 : Inport  OutDataTypeStr=fixdt(0, 2, 0)  PortDimensions=1  SampleTime=2.5e-07
  Extract Bits2 : simulink/Logic and Bit Operations/Extract Bits  bitsToExtract=Upper half  numBits=8  bitIdxRange=[32 63]  outScalingMode=Treat bit field as an integer
  Extract Bits3 : simulink/Logic and Bit Operations/Extract Bits  bitsToExtract=Lower half  numBits=8  bitIdxRange=[32 63]  outScalingMode=Treat bit field as an integer
  Mux1 : Mux  Inputs=2
  Out1 : Outport  SampleTime=2.5e-07
  wires:
  In1/1 -> Extract Bits2/1, Extract Bits3/1
  Extract Bits3/1 -> Mux1/2
  Extract Bits2/1 -> Mux1/1
  Mux1/1 -> Out1/1

== system gm_soc_dvbs2_fpga/DVBS2/DVBS2 TxRx/DVB-S2 HDL Receiver/Synchronizer and PL Header Decoder/PL Header Recovery/PL Header Decoder/ML Decoder/Integer to Bit Convertor/For Each Subsystem3_instance7 ==
  note: For Each
  In1 : Inport  OutDataTypeStr=fixdt(0, 2, 0)  PortDimensions=1  SampleTime=2.5e-07
  Extract Bits2 : simulink/Logic and Bit Operations/Extract Bits  bitsToExtract=Upper half  numBits=8  bitIdxRange=[32 63]  outScalingMode=Treat bit field as an integer
  Extract Bits3 : simulink/Logic and Bit Operations/Extract Bits  bitsToExtract=Lower half  numBits=8  bitIdxRange=[32 63]  outScalingMode=Treat bit field as an integer
  Mux1 : Mux  Inputs=2
  Out1 : Outport  SampleTime=2.5e-07
  wires:
  In1/1 -> Extract Bits2/1, Extract Bits3/1
  Extract Bits2/1 -> Mux1/1
  Extract Bits3/1 -> Mux1/2
  Mux1/1 -> Out1/1

== system gm_soc_dvbs2_fpga/DVBS2/DVBS2 TxRx/DVB-S2 HDL Receiver/Synchronizer and PL Header Decoder/PL Header Recovery/PL Header Decoder/ML Decoder/Integer to Bit Convertor/For Each Subsystem3_instance8 ==
  note: For Each
  In1 : Inport  OutDataTypeStr=fixdt(0, 2, 0)  PortDimensions=1  SampleTime=2.5e-07
  Extract Bits2 : simulink/Logic and Bit Operations/Extract Bits  bitsToExtract=Upper half  numBits=8  bitIdxRange=[32 63]  outScalingMode=Treat bit field as an integer
  Extract Bits3 : simulink/Logic and Bit Operations/Extract Bits  bitsToExtract=Lower half  numBits=8  bitIdxRange=[32 63]  outScalingMode=Treat bit field as an integer
  Mux1 : Mux  Inputs=2
  Out1 : Outport  SampleTime=2.5e-07
  wires:
  Extract Bits3/1 -> Mux1/2
  In1/1 -> Extract Bits2/1, Extract Bits3/1
  Extract Bits2/1 -> Mux1/1
  Mux1/1 -> Out1/1

== system gm_soc_dvbs2_fpga/DVBS2/DVBS2 TxRx/DVB-S2 HDL Receiver/Synchronizer and PL Header Decoder/PL Header Recovery/PL Header Decoder/ML Decoder/Integer to Bit Convertor/For Each Subsystem3_instance9 ==
  note: For Each
  In1 : Inport  OutDataTypeStr=fixdt(0, 2, 0)  PortDimensions=1  SampleTime=2.5e-07
  Extract Bits2 : simulink/Logic and Bit Operations/Extract Bits  bitsToExtract=Upper half  numBits=8  bitIdxRange=[32 63]  outScalingMode=Treat bit field as an integer
  Extract Bits3 : simulink/Logic and Bit Operations/Extract Bits  bitsToExtract=Lower half  numBits=8  bitIdxRange=[32 63]  outScalingMode=Treat bit field as an integer
  Mux1 : Mux  Inputs=2
  Out1 : Outport  SampleTime=2.5e-07
  wires:
  In1/1 -> Extract Bits3/1, Extract Bits2/1
  Extract Bits3/1 -> Mux1/2
  Extract Bits2/1 -> Mux1/1
  Mux1/1 -> Out1/1

== system gm_soc_dvbs2_fpga/DVBS2/DVBS2 TxRx/DVB-S2 HDL Receiver/Synchronizer and PL Header Decoder/PL Header Recovery/PL Header Decoder/ML Decoder/Integer to Bit Convertor/For Each Subsystem4_instance1 ==
  note: For Each
  In1 : Inport  OutDataTypeStr=uint16  PortDimensions=1  SampleTime=2.5e-07
  Extract Bits2 : simulink/Logic and Bit Operations/Extract Bits  bitsToExtract=Upper half  numBits=8  bitIdxRange=[32 63]  outScalingMode=Treat bit field as an integer
  Extract Bits3 : simulink/Logic and Bit Operations/Extract Bits  bitsToExtract=Lower half  numBits=8  bitIdxRange=[32 63]  outScalingMode=Treat bit field as an integer
  Mux1 : Mux  Inputs=2
  Out1 : Outport  SampleTime=2.5e-07
  wires:
  Extract Bits3/1 -> Mux1/2
  In1/1 -> Extract Bits2/1, Extract Bits3/1
  Extract Bits2/1 -> Mux1/1
  Mux1/1 -> Out1/1

== system gm_soc_dvbs2_fpga/DVBS2/DVBS2 TxRx/DVB-S2 HDL Receiver/Synchronizer and PL Header Decoder/PL Header Recovery/PL Header Decoder/ML Decoder/Integer to Bit Convertor/For Each Subsystem4_instance2 ==
  note: For Each
  In1 : Inport  OutDataTypeStr=uint16  PortDimensions=1  SampleTime=2.5e-07
  Extract Bits2 : simulink/Logic and Bit Operations/Extract Bits  bitsToExtract=Upper half  numBits=8  bitIdxRange=[32 63]  outScalingMode=Treat bit field as an integer
  Extract Bits3 : simulink/Logic and Bit Operations/Extract Bits  bitsToExtract=Lower half  numBits=8  bitIdxRange=[32 63]  outScalingMode=Treat bit field as an integer
  Mux1 : Mux  Inputs=2
  Out1 : Outport  SampleTime=2.5e-07
  wires:
  In1/1 -> Extract Bits2/1, Extract Bits3/1
  Extract Bits3/1 -> Mux1/2
  Extract Bits2/1 -> Mux1/1
  Mux1/1 -> Out1/1

== system gm_soc_dvbs2_fpga/DVBS2/DVBS2 TxRx/DVB-S2 HDL Receiver/Synchronizer and PL Header Decoder/PL Header Recovery/PL Header Decoder/ML Decoder/Integer to Bit Convertor/For Each Subsystem5_instance1 ==
  note: For Each
  In1 : Inport  OutDataTypeStr=uint8  PortDimensions=1  SampleTime=2.5e-07
  Extract Bits2 : simulink/Logic and Bit Operations/Extract Bits  bitsToExtract=Upper half  numBits=8  bitIdxRange=[32 63]  outScalingMode=Treat bit field as an integer
  Extract Bits3 : simulink/Logic and Bit Operations/Extract Bits  bitsToExtract=Lower half  numBits=8  bitIdxRange=[32 63]  outScalingMode=Treat bit field as an integer
  Mux1 : Mux  Inputs=2
  Out1 : Outport  SampleTime=2.5e-07
  wires:
  Extract Bits3/1 -> Mux1/2
  In1/1 -> Extract Bits2/1, Extract Bits3/1
  Extract Bits2/1 -> Mux1/1
  Mux1/1 -> Out1/1

== system gm_soc_dvbs2_fpga/DVBS2/DVBS2 TxRx/DVB-S2 HDL Receiver/Synchronizer and PL Header Decoder/PL Header Recovery/PL Header Decoder/ML Decoder/Integer to Bit Convertor/For Each Subsystem5_instance2 ==
  note: For Each
  In1 : Inport  OutDataTypeStr=uint8  PortDimensions=1  SampleTime=2.5e-07
  Extract Bits2 : simulink/Logic and Bit Operations/Extract Bits  bitsToExtract=Upper half  numBits=8  bitIdxRange=[32 63]  outScalingMode=Treat bit field as an integer
  Extract Bits3 : simulink/Logic and Bit Operations/Extract Bits  bitsToExtract=Lower half  numBits=8  bitIdxRange=[32 63]  outScalingMode=Treat bit field as an integer
  Mux1 : Mux  Inputs=2
  Out1 : Outport  SampleTime=2.5e-07
  wires:
  In1/1 -> Extract Bits2/1, Extract Bits3/1
  Extract Bits3/1 -> Mux1/2
  Extract Bits2/1 -> Mux1/1
  Mux1/1 -> Out1/1

== system gm_soc_dvbs2_fpga/DVBS2/DVBS2 TxRx/DVB-S2 HDL Receiver/Synchronizer and PL Header Decoder/PL Header Recovery/PL Header Decoder/ML Decoder/Integer to Bit Convertor/For Each Subsystem5_instance3 ==
  note: For Each
  In1 : Inport  OutDataTypeStr=uint8  PortDimensions=1  SampleTime=2.5e-07
  Extract Bits2 : simulink/Logic and Bit Operations/Extract Bits  bitsToExtract=Upper half  numBits=8  bitIdxRange=[32 63]  outScalingMode=Treat bit field as an integer
  Extract Bits3 : simulink/Logic and Bit Operations/Extract Bits  bitsToExtract=Lower half  numBits=8  bitIdxRange=[32 63]  outScalingMode=Treat bit field as an integer
  Mux1 : Mux  Inputs=2
  Out1 : Outport  SampleTime=2.5e-07
  wires:
  In1/1 -> Extract Bits2/1, Extract Bits3/1
  Extract Bits2/1 -> Mux1/1
  Extract Bits3/1 -> Mux1/2
  Mux1/1 -> Out1/1

== system gm_soc_dvbs2_fpga/DVBS2/DVBS2 TxRx/DVB-S2 HDL Receiver/Synchronizer and PL Header Decoder/PL Header Recovery/PL Header Decoder/ML Decoder/Integer to Bit Convertor/For Each Subsystem5_instance4 ==
  note: For Each
  In1 : Inport  OutDataTypeStr=uint8  PortDimensions=1  SampleTime=2.5e-07
  Extract Bits2 : simulink/Logic and Bit Operations/Extract Bits  bitsToExtract=Upper half  numBits=8  bitIdxRange=[32 63]  outScalingMode=Treat bit field as an integer
  Extract Bits3 : simulink/Logic and Bit Operations/Extract Bits  bitsToExtract=Lower half  numBits=8  bitIdxRange=[32 63]  outScalingMode=Treat bit field as an integer
  Mux1 : Mux  Inputs=2
  Out1 : Outport  SampleTime=2.5e-07
  wires:
  Extract Bits3/1 -> Mux1/2
  In1/1 -> Extract Bits2/1, Extract Bits3/1
  Extract Bits2/1 -> Mux1/1
  Mux1/1 -> Out1/1

== system gm_soc_dvbs2_fpga/DVBS2/DVBS2 TxRx/DVB-S2 HDL Receiver/Synchronizer and PL Header Decoder/PL Header Recovery/PL Header Decoder/ML Decoder/Integer to Bit Convertor/For Each Subsystem6_instance1 ==
  note: For Each
  In1 : Inport  OutDataTypeStr=fixdt(0, 4, 0)  PortDimensions=1  SampleTime=2.5e-07
  Extract Bits2 : simulink/Logic and Bit Operations/Extract Bits  bitsToExtract=Upper half  numBits=8  bitIdxRange=[32 63]  outScalingMode=Treat bit field as an integer
  Extract Bits3 : simulink/Logic and Bit Operations/Extract Bits  bitsToExtract=Lower half  numBits=8  bitIdxRange=[32 63]  outScalingMode=Treat bit field as an integer
  Mux1 : Mux  Inputs=2
  Out1 : Outport  SampleTime=2.5e-07
  wires:
  Extract Bits3/1 -> Mux1/2
  In1/1 -> Extract Bits2/1, Extract Bits3/1
  Extract Bits2/1 -> Mux1/1
  Mux1/1 -> Out1/1

== system gm_soc_dvbs2_fpga/DVBS2/DVBS2 TxRx/DVB-S2 HDL Receiver/Synchronizer and PL Header Decoder/PL Header Recovery/PL Header Decoder/ML Decoder/Integer to Bit Convertor/For Each Subsystem6_instance2 ==
  note: For Each
  In1 : Inport  OutDataTypeStr=fixdt(0, 4, 0)  PortDimensions=1  SampleTime=2.5e-07
  Extract Bits2 : simulink/Logic and Bit Operations/Extract Bits  bitsToExtract=Upper half  numBits=8  bitIdxRange=[32 63]  outScalingMode=Treat bit field as an integer
  Extract Bits3 : simulink/Logic and Bit Operations/Extract Bits  bitsToExtract=Lower half  numBits=8  bitIdxRange=[32 63]  outScalingMode=Treat bit field as an integer
  Mux1 : Mux  Inputs=2
  Out1 : Outport  SampleTime=2.5e-07
  wires:
  In1/1 -> Extract Bits2/1, Extract Bits3/1
  Extract Bits3/1 -> Mux1/2
  Extract Bits2/1 -> Mux1/1
  Mux1/1 -> Out1/1

== system gm_soc_dvbs2_fpga/DVBS2/DVBS2 TxRx/DVB-S2 HDL Receiver/Synchronizer and PL Header Decoder/PL Header Recovery/PL Header Decoder/ML Decoder/Integer to Bit Convertor/For Each Subsystem6_instance3 ==
  note: For Each
  In1 : Inport  OutDataTypeStr=fixdt(0, 4, 0)  PortDimensions=1  SampleTime=2.5e-07
  Extract Bits2 : simulink/Logic and Bit Operations/Extract Bits  bitsToExtract=Upper half  numBits=8  bitIdxRange=[32 63]  outScalingMode=Treat bit field as an integer
  Extract Bits3 : simulink/Logic and Bit Operations/Extract Bits  bitsToExtract=Lower half  numBits=8  bitIdxRange=[32 63]  outScalingMode=Treat bit field as an integer
  Mux1 : Mux  Inputs=2
  Out1 : Outport  SampleTime=2.5e-07
  wires:
  In1/1 -> Extract Bits2/1, Extract Bits3/1
  Extract Bits2/1 -> Mux1/1
  Extract Bits3/1 -> Mux1/2
  Mux1/1 -> Out1/1

== system gm_soc_dvbs2_fpga/DVBS2/DVBS2 TxRx/DVB-S2 HDL Receiver/Synchronizer and PL Header Decoder/PL Header Recovery/PL Header Decoder/ML Decoder/Integer to Bit Convertor/For Each Subsystem6_instance4 ==
  note: For Each
  In1 : Inport  OutDataTypeStr=fixdt(0, 4, 0)  PortDimensions=1  SampleTime=2.5e-07
  Extract Bits2 : simulink/Logic and Bit Operations/Extract Bits  bitsToExtract=Upper half  numBits=8  bitIdxRange=[32 63]  outScalingMode=Treat bit field as an integer
  Extract Bits3 : simulink/Logic and Bit Operations/Extract Bits  bitsToExtract=Lower half  numBits=8  bitIdxRange=[32 63]  outScalingMode=Treat bit field as an integer
  Mux1 : Mux  Inputs=2
  Out1 : Outport  SampleTime=2.5e-07
  wires:
  Extract Bits3/1 -> Mux1/2
  In1/1 -> Extract Bits2/1, Extract Bits3/1
  Extract Bits2/1 -> Mux1/1
  Mux1/1 -> Out1/1
